simulink model "INTER_IIT_2ndorder_without_noise_DSM"  (R2024b)
settings: Solver=VariableStepAuto  StartTime=0.0  StopTime=10.0  RelTol=1e-3
undefined symbols (not defined in the file): DiscIntNeverNeededParam
settings Model: Creator=somya  LastModifiedBy=rishi

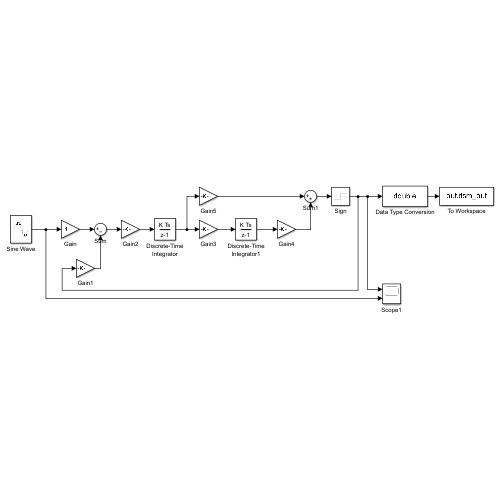
[thumbnail: Simulink's stored preview of the top-level diagram]
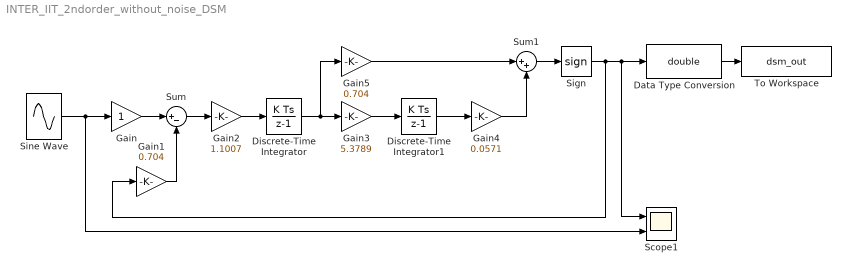
== system INTER_IIT_2ndorder_without_noise_DSM ==
  Data Type Conversion : DataTypeConversion  OutDataTypeStr=double  SaturateOnIntegerOverflow=off  RndMeth=Floor
  Discrete-Time Integrator : DiscreteIntegrator  SampleTime=-1  ICPrevOutput=DiscIntNeverNeededParam  ICPrevScaledInput=DiscIntNeverNeededParam
  Discrete-Time Integrator1 : DiscreteIntegrator  SampleTime=-1  ICPrevOutput=DiscIntNeverNeededParam  ICPrevScaledInput=DiscIntNeverNeededParam
  Gain : Gain
  Gain1 : Gain  Gain=0.704
  Gain2 : Gain  Gain=1.1007
  Gain3 : Gain  Gain=5.3789
  Gain4 : Gain  Gain=0.0571
  Gain5 : Gain  Gain=0.704
  Scope1 : Scope  NumInputPorts=2
  Sign : Signum
  Sine Wave : Sin  Amplitude=0.5  Frequency=306.796157  Samples=150000  SampleTime=1.22e-7  VectorParams1D=off
  Sum : Sum  Inputs=|+-
  Sum1 : Sum  Inputs=|++
  To Workspace : ToWorkspace  VariableName=dsm_out  SampleTime=-1
  wires:
  Gain5/1 -> Sum1/1
  Gain3/1 -> Discrete-Time Integrator1/1
  Data Type Conversion/1 -> To Workspace/1
  Sum1/1 -> Sign/1
  Sign/1 -> Data Type Conversion/1, Scope1/1, Gain1/1
  Gain2/1 -> Discrete-Time Integrator/1
  Discrete-Time Integrator1/1 -> Gain4/1
  Gain1/1 -> Sum/2
  Gain4/1 -> Sum1/2
  Sum/1 -> Gain2/1
  Discrete-Time Integrator/1 -> Gain3/1, Gain5/1
  Gain/1 -> Sum/1
  Sine Wave/1 -> Scope1/2, Gain/1
